simulink model "model"  (R2023a)
settings: Solver=VariableStepAuto  StartTime=0.0  StopTime=10.0  RelTol=1e-3
libraries: BatteryCurrentManagement x2
settings Model: Creator=Pedro  LastModifiedBy=Pedro

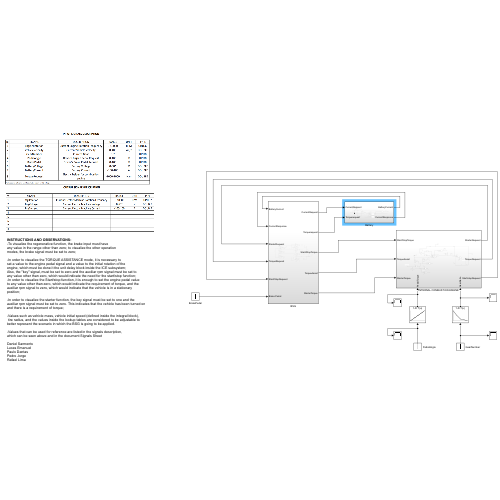
[thumbnail: Simulink's stored preview of the top-level diagram]
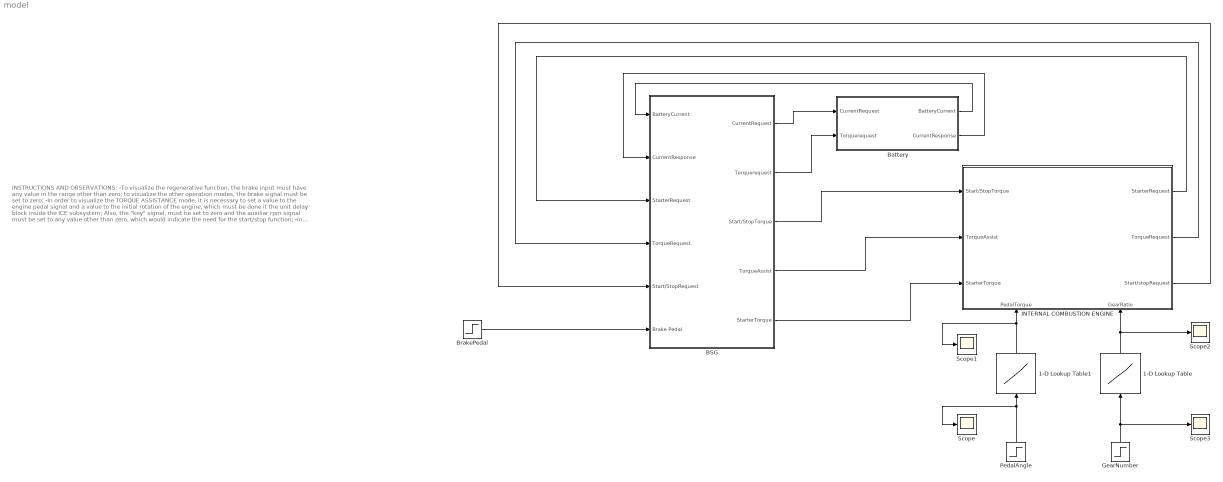
== system model ==
  note: INSTRUCTIONS AND OBSERVATIONS:
      | -To visualize the regenerative function, the brake input must have
      | any value in the range other than zero; to visualize the other operation
      | modes, the brake signal must be set to zero;
      |
      | -In order to visualize the TORQUE ASSISTANCE mode, it is necessary to
      | set a value to the engine pedal signal and a value to the initial rotation of the
      | engine, which must be done it the unit delay block inside the ICE subsystem;
      | Also, the "key" signal, must be set to zero and the auxiliar rpm signal must be set to
      | any value other than zero, which would indicate the need for the start/stop function;
      | -In order to visualize the Start/stop function, it is enough to set the engine pedal value
      | to any value other than zero, which would indicate the requirement of torque, and the
      | auxiliar rpm signal to zero, which would indicate that the vehicle is in a stationary
      | position;
      |
      | -In order to visualize the starter function, the key signal must be set to one and the
      | auxiliar rpm signal must be set to zero. This indicates that the vehicle has been turned on
      | and there is a requirement of torque;
      |
      | -Values such as vehicle mass, vehicle initial speed (defined inside the integral block),
      | tire radius, and the values inside the lookup tables are considered to be adjustable to
      | better represent the scenario in which the BSG is going to be applied.
      |
      | -Values that can be used for reference are listed in the signals description,
      | which can be seen above and in the document Signals Sheet
      |
      | Daniel Sarmento
      | Lucas Emanuel
      | Paulo Dantas
      | Pedro Jorge
      | Rafael Lima
  1-D Lookup Table : Lookup_n-D  NumberOfTableDimensions=1  BreakpointsForDimension1=[1 2 3 4 5]  Table=[3 2 1.2 1 0.8]  InternalRulePriority=Speed  RndMeth=Simplest
  1-D Lookup Table1 : Lookup_n-D  NumberOfTableDimensions=1  BreakpointsForDimension1=|  Table=|  InternalRulePriority=Speed  RndMeth=Simplest
      BreakpointsForDimension1=|
      | [0
      | 0.5
      | 1
      | 1.5
      | 2
      | 2.5
      | 3
      | 3.5
      | 4
      | 4.5
      | 5
      | 5.5
      | 6
      | 6.5
      | 7
      | 7.5
      | 8
      | 8.5
      | 9
      | 9.5
      | 10
      | 10.5
      | 11
      | 11.5
      | 12
      | 12.5
      | 13
      | 13.5
      | 14
      | 14.5
      | 15
      | 15.5
      | 16
      | 16.5
      | 17
      | 17.5
      | 18
      | 18.5
      | 19
      | 19.5
      | 20
      | 20.5
      | 21
      | 21.5
      | 22
      | 22.5
      | 23
      | 23.5
      | 24
      | 24.5
      | 25
      | 25.5
      | 26
      | 26.5
      | 27
      | 27.5
      | 28
      | 28.5
      | 29
      | 29.5
      | 30
      | 30.5
      | 31
      | 31.5
      | 32
      | 32.5
      | 33
      | 33.5
      | 34
      | 34.5
      | 35
      | 35.5
      | 36
      | 36.5
      | 37
      | 37.5
      | 38
      | 38.5
      | 39
      | 39.5
      | 40
      | 40.5
      | 41
      | 41.5
      | 42
      | 42.5
      | 43
      | 43.5
      | 44
      | 44.5
      | 45
      | 45.5
      | 46
      | 46.5
      | 47
      | 47.5
      | 48
      | 48.5
      | 49
      | 49.5
      | 50
      | 50.5
      | 51
      | 51.5
      | 52
      | 52.5
      | 53
      | 53.5
      | 54
      | 54.5
      | 55
      | 55.5
      | 56
      | 56.5
      | 57
      | 57.5
      | 58
      | 58.5
      | 59
      | 59.5
      | 60
      | 60.5
      | 61
      | 61.5
      | 62
      | 62.5
      | 63
      | 63.5
      | 64
      | 64.5
      | 65
      | 65.5
      | 66
      | 66.5
      | 67
      | 67.5
      | 68
      | 68.5
      | 69
      | 69.5
      | 70
      | 70.5
      | 71
      | 71.5
      | 72
      | 72.5
      | 73
      | 73.5
      | 74
      | 74.5
      | 75
      | 75.5
      | 76
      | 76.5
      | 77
      | 77.5
      | 78
      | 78.5
      | 79
      | 79.5
      | 80
      | 80.5
      | 81
      | 81.5
      | 82
      | 82.5
      | 83
      | 83.5
      | 84
      | 84.5
      | 85
      | 85.5
      | 86
      | 86.5
      | 87
      | 87.5
      | 88
      | 88.5
      | 89
      | 89.5
      | 90
      | 90.5
      | 91
      | 91.5
      | 92
      | 92.5
      | 93
      | 93.5
      | 94
      | 94.5
      | 95
      | 95.5
      | 96
      | 96.5
      | 97
      | 97.5
      | 98
      | 98.5
      | 99
      | 99.5
      | 100
      | ]
      Table=|
      | [0
      | 2
      | 4
      | 6
      | 8
      | 10
      | 12
      | 14
      | 16
      | 18
      | 20
      | 22
      | 24
      | 26
      | 28
      | 30
      | 32
      | 34
      | 36
      | 38
      | 40
      | 42
      | 44
      | 46
      | 48
      | 50
      | 52
      | 54
      | 56
      | 58
      | 60
      | 62
      | 64
      | 66
      | 68
      | 70
      | 72
      | 74
      | 76
      | 78
      | 80
      | 82
      | 84
      | 86
      | 88
      | 90
      | 92
      | 94
      | 96
      | 98
      | 100
      | 102
      | 104
      | 106
      | 108
      | 110
      | 112
      | 114
      | 116
      | 118
      | 120
      | 122
      | 124
      | 126
      | 128
      | 130
      | 132
      | 134
      | 136
      | 138
      | 140
      | 142
      | 144
      | 146
      | 148
      | 150
      | 152
      | 154
      | 156
      | 158
      | 160
      | 162
      | 164
      | 166
      | 168
      | 170
      | 172
      | 174
      | 176
      | 178
      | 180
      | 182
      | 184
      | 186
      | 188
      | 190
      | 192
      | 194
      | 196
      | 198
      | 200
      | 202
      | 204
      | 206
      | 208
      | 210
      | 212
      | 214
      | 216
      | 218
      | 220
      | 222
      | 224
      | 226
      | 228
      | 230
      | 232
      | 234
      | 236
      | 238
      | 240
      | 242
      | 244
      | 246
      | 248
      | 250
      | 252
      | 254
      | 256
      | 258
      | 260
      | 262
      | 264
      | 266
      | 268
      | 270
      | 272
      | 274
      | 276
      | 278
      | 280
      | 282
      | 284
      | 286
      | 288
      | 290
      | 292
      | 294
      | 296
      | 298
      | 300
      | 302
      | 304
      | 306
      | 308
      | 310
      | 312
      | 314
      | 316
      | 318
      | 320
      | 322
      | 324
      | 326
      | 328
      | 330
      | 332
      | 334
      | 336
      | 338
      | 340
      | 342
      | 344
      | 346
      | 348
      | 350
      | 352
      | 354
      | 356
      | 358
      | 360
      | 362
      | 364
      | 366
      | 368
      | 370
      | 372
      | 374
      | 376
      | 378
      | 380
      | 382
      | 384
      | 386
      | 388
      | 390
      | 392
      | 394
      | 396
      | 398
      | 400]
  BSG : Subsystem
  Battery : Subsystem
  BrakePedal : Step  Before=5  After=5  SampleTime=0
  GearNumber : Step  Before=3  After=3  SampleTime=0
  INTERNAL COMBUSTION ENGINE : Subsystem
      settings: PortSchema="{\"entries\":[{\"content\":{\"sides\":[{\"content\":{\"connectorIds\":[\"In1\",\"In2\",\"In3\"]},\"type\":\"ConnectorPlacement.EquallySpacedRectSide\",\"uuid\":\"ce092393-4b5e-4455-aba9-0cf9705a5882\"},{\"content\":{\"connectorIds\":[\"Out1\",\"Out2\",\"Out3\"],\"side\":\"RIGHT\"},\"type\":\"ConnectorPlacement.EquallySpacedRectSide\",\"uuid\":\"39f1620d-f19f-4d17-9a2c-1204b4040c22\"},{\"content\":{\"side\":\"TOP\"},\"type\":\"ConnectorPlacement.EquallySpacedRectSide\",\"uuid\":\"940edc2a-8e4d-4800-9ba5-7e24d0f8ee78\"},{\"content\":{\"connectorIds\":[\"In4\",\"In5\"],\"side\":\"BOTTOM\"},\"type\":\"ConnectorPlacement.EquallySpacedRectSide\",\"uuid\":\"a8c92029-a525-4a44-9138-e7028dc0182e\"}]},\"type\":\"ConnectorPlacement.EquallySpacedConnector\",\"uuid\":\"b09c41f2-a1e2-4cd1-915a-dc8e84f252cd\"}],\"packageUris\":[\"http://schema.mathworks.com/mf0/Connector/R2020b\"],\"version\":\"1.0\"}"
  PedalAngle : Step  Before=10  After=10  SampleTime=0
  Scope{,1..3} (4 alike) : Scope
  wires:
  Battery/2(CurrentResponse) -> BSG/2(CurrentResponse)
  PedalAngle/1 -> Scope/1, 1-D Lookup Table1/1
  BrakePedal/1 -> BSG/6(Brake Pedal)
  INTERNAL COMBUSTION ENGINE/2(TorqueRequest) -> BSG/4(TorqueRequest)
  INTERNAL COMBUSTION ENGINE/3(Start/stopRequest) -> BSG/5(Start/StopRequest)
  INTERNAL COMBUSTION ENGINE/1(StarterRequest) -> BSG/3(StarterRequest)
  GearNumber/1 -> 1-D Lookup Table/1, Scope3/1
  1-D Lookup Table/1 -> Scope2/1, INTERNAL COMBUSTION ENGINE/5(GearRatio)
  BSG/3(Start/StopTorque) -> INTERNAL COMBUSTION ENGINE/1(Start/StopTorque)
  BSG/4(TorqueAssist) -> INTERNAL COMBUSTION ENGINE/2(TorqueAssist)
  BSG/5(StarterTorque) -> INTERNAL COMBUSTION ENGINE/3(StarterTorque)
  Battery/1(BatteryCurrent) -> BSG/1(BatteryCurrent)
  BSG/1(CurrentRequest) -> Battery/1(CurrentRequest)
  1-D Lookup Table1/1 -> Scope1/1, INTERNAL COMBUSTION ENGINE/4(PedalTorque)
  BSG/2(Torquerequest) -> Battery/2(Torquerequest)

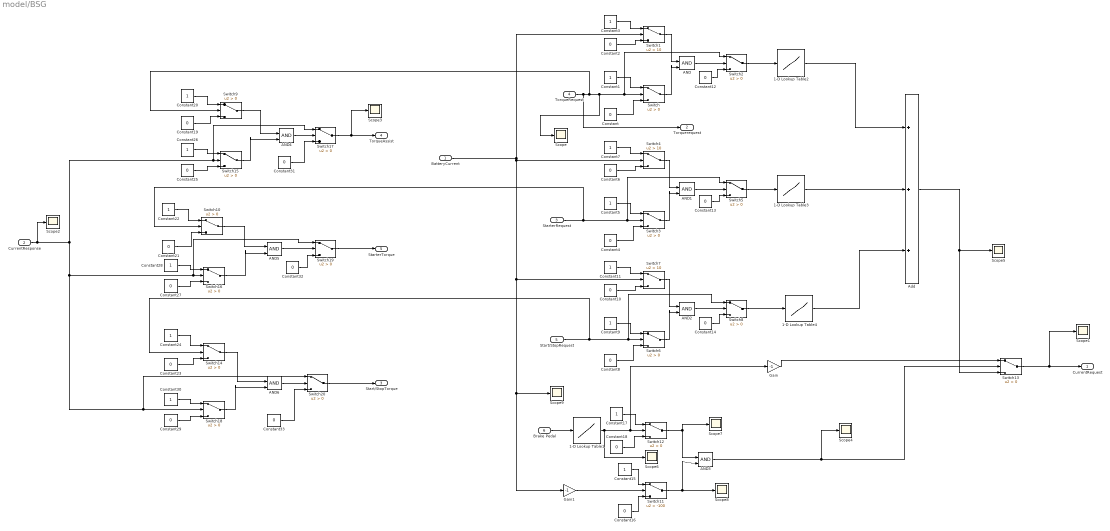
== system model/BSG ==
  BatteryCurrent : Inport
  CurrentResponse : Inport  Port=2
  StarterRequest : Inport  Port=3
  TorqueRequest : Inport  Port=4
  Start/StopRequest : Inport  Port=5
  Brake Pedal : Inport  Port=6
  1-D Lookup Table1 : Lookup_n-D  NumberOfTableDimensions=1  BreakpointsForDimension1=|  Table=|  InternalRulePriority=Speed  RndMeth=Simplest
      | [0
      | 5
      | 10
      | 15
      | 20
      | 25
      | 30
      | 35
      | 40
      | 45
      | 50
      | 55
      | 60
      | 65
      | 70
      | 75
      | 80
      | 85
      | 90
      | 95
      | 100
      | ]
      | [0
      | 5
      | 10
      | 15
      | 20
      | 25
      | 30
      | 35
      | 40
      | 45
      | 50
      | 55
      | 60
      | 65
      | 70
      | 75
      | 80
      | 85
      | 90
      | 95
      | 100
      | ]
  1-D Lookup Table2 : Lookup_n-D  NumberOfTableDimensions=1  BreakpointsForDimension1=|  Table=|  InternalRulePriority=Speed  RndMeth=Simplest
      | [0
      | 10
      | 20
      | 30
      | 40
      | 50
      | 60
      | 70
      | 80
      | 90
      | 100
      | 110
      | 120
      | 130
      | 140
      | 150
      | 160
      | 170
      | 180
      | 190
      | 200
      | 210
      | 220
      | 230
      | 240
      | 250
      | 260
      | 270
      | 280
      | 290
      | 300
      | ]
      | [0
      | 1.7
      | 4.4
      | 7.1
      | 9.8
      | 12.5
      | 15.2
      | 17.9
      | 20.6
      | 23.3
      | 26
      | 28.7
      | 31.4
      | 34.1
      | 36.8
      | 39.5
      | 42.2
      | 44.9
      | 47.6
      | 50.3
      | 53
      | 55.7
      | 58.4
      | 61.1
      | 63.8
      | 66.5
      | 69.2
      | 71.9
      | 74.6
      | 77.3
      | 80
      | ]
  1-D Lookup Table3 : Lookup_n-D  NumberOfTableDimensions=1  BreakpointsForDimension1=|  Table=|  InternalRulePriority=Speed  RndMeth=Simplest
      | [0
      | 10
      | 20
      | 30
      | 40
      | 50
      | 60
      | 70
      | 80
      | 90
      | 100
      | 110
      | 120
      | 130
      | 140
      | 150
      | 160
      | 170
      | 180
      | 190
      | 200
      | 210
      | 220
      | 230
      | 240
      | 250
      | 260
      | 270
      | 280
      | 290
      | 300
      | ]
      | [0
      | 1.7
      | 4.4
      | 7.1
      | 9.8
      | 12.5
      | 15.2
      | 17.9
      | 20.6
      | 23.3
      | 26
      | 28.7
      | 31.4
      | 34.1
      | 36.8
      | 39.5
      | 42.2
      | 44.9
      | 47.6
      | 50.3
      | 53
      | 55.7
      | 58.4
      | 61.1
      | 63.8
      | 66.5
      | 69.2
      | 71.9
      | 74.6
      | 77.3
      | 80
      | ]
  1-D Lookup Table4 : Lookup_n-D  NumberOfTableDimensions=1  BreakpointsForDimension1=|  Table=|  InternalRulePriority=Speed  RndMeth=Simplest
      | [0
      | 10
      | 20
      | 30
      | 40
      | 50
      | 60
      | 70
      | 80
      | 90
      | 100
      | 110
      | 120
      | 130
      | 140
      | 150
      | 160
      | 170
      | 180
      | 190
      | 200
      | 210
      | 220
      | 230
      | 240
      | 250
      | 260
      | 270
      | 280
      | 290
      | 300
      | ]
      | [0
      | 1.7
      | 4.4
      | 7.1
      | 9.8
      | 12.5
      | 15.2
      | 17.9
      | 20.6
      | 23.3
      | 26
      | 28.7
      | 31.4
      | 34.1
      | 36.8
      | 39.5
      | 42.2
      | 44.9
      | 47.6
      | 50.3
      | 53
      | 55.7
      | 58.4
      | 61.1
      | 63.8
      | 66.5
      | 69.2
      | 71.9
      | 74.6
      | 77.3
      | 80
      | ]
  AND{,1..6} (7 alike) : Logic  IconShape=distinctive  AllPortsSameDT=off  OutDataTypeStr=boolean
  Add : Sum  Inputs=+++
  Constant{,2,4,6,8,10,12..14,16,18..19,21,23,25,27,29,31..33} (20 alike) : Constant  Value=0
  Constant{1,3,5,7,9,11,15,17,20,22,24,26,28,30} (14 alike) : Constant
  Gain : Gain  Gain=-1
  Gain1 : Gain  Gain=-1
  Scope{,1..9} (10 alike) : Scope
  Switch{,2..3,5..6,8..10,12..20} (17 alike) : Switch  Criteria=u2 > Threshold  SaturateOnIntegerOverflow=off  InputSameDT=off
  Switch1 : Switch  Criteria=u2 > Threshold  Threshold=10  SaturateOnIntegerOverflow=off  InputSameDT=off
  Switch11 : Switch  Criteria=u2 > Threshold  Threshold=-100  SaturateOnIntegerOverflow=off  InputSameDT=off
  Switch4 : Switch  Criteria=u2 > Threshold  Threshold=10  SaturateOnIntegerOverflow=off  InputSameDT=off
  Switch7 : Switch  Criteria=u2 > Threshold  Threshold=10  SaturateOnIntegerOverflow=off  InputSameDT=off
  CurrentRequest : Outport
  Torquerequest : Outport  Port=2
  Start/StopTorque : Outport  Port=3
  TorqueAssist : Outport  Port=4
  StarterTorque : Outport  Port=5
  wires:
  Constant14/1 -> Switch8/3
  Constant11/1 -> Switch7/1
  Constant8/1 -> Switch6/3
  Constant6/1 -> Switch4/3
  Constant10/1 -> Switch7/3
  AND1/1 -> Switch5/2
  Constant12/1 -> Switch2/3
  Switch7/1 -> AND2/1
  StarterRequest/1 -> Switch10/2, Switch5/1, Switch3/2
  Constant13/1 -> Switch5/3
  AND2/1 -> Switch8/2
  AND/1 -> Switch2/2
  Constant4/1 -> Switch3/3
  Constant2/1 -> Switch1/3
  Constant5/1 -> Switch3/1
  Switch6/1 -> AND2/2
  Switch4/1 -> AND1/1
  Constant3/1 -> Switch1/1
  Constant/1 -> Switch/3
  Switch/1 -> AND/2
  1-D Lookup Table2/1 -> Add/1
  Constant1/1 -> Switch/1
  Switch3/1 -> AND1/2
  Switch5/1 -> 1-D Lookup Table3/1
  TorqueRequest/1 -> Torquerequest/1, Switch9/2, Scope/1, Switch2/1, Switch/2
  Start/StopRequest/1 -> Switch14/2, Switch8/1, Switch6/2
  Constant7/1 -> Switch4/1
  Constant9/1 -> Switch6/1
  BatteryCurrent/1 -> Gain1/1, Scope9/1, Switch7/2, Switch4/2, Switch1/2
  Switch2/1 -> 1-D Lookup Table2/1
  Switch1/1 -> AND/1
  Switch8/1 -> 1-D Lookup Table4/1
  Brake Pedal/1 -> 1-D Lookup Table1/1
  Constant15/1 -> Switch11/1
  Constant16/1 -> Switch11/3
  Gain1/1 -> Switch11/2
  1-D Lookup Table1/1 -> Scope6/1, Gain/1, Switch12/2
  Constant17/1 -> Switch12/1
  Constant18/1 -> Switch12/3
  Switch12/1 -> AND3/1, Scope7/1
  Switch11/1 -> AND3/2, Scope8/1
  Gain/1 -> Switch13/1
  1-D Lookup Table3/1 -> Add/2
  1-D Lookup Table4/1 -> Add/3
  Add/1 -> Switch13/3, Scope5/1
  Switch13/1 -> Scope1/1, CurrentRequest/1
  Constant19/1 -> Switch9/3
  Constant20/1 -> Switch9/1
  Constant22/1 -> Switch10/1
  Constant21/1 -> Switch10/3
  Constant23/1 -> Switch14/3
  Constant24/1 -> Switch14/1
  Constant25/1 -> Switch15/3
  CurrentResponse/1 -> Scope2/1, Switch20/1, Switch18/2, Switch19/1, Switch16/2, Switch17/1, Switch15/2
  Constant26/1 -> Switch15/1
  Constant27/1 -> Switch16/3
  Constant28/1 -> Switch16/1
  Constant29/1 -> Switch18/3
  Constant30/1 -> Switch18/1
  Switch9/1 -> AND4/1
  Switch15/1 -> AND4/2
  Switch10/1 -> AND5/1
  Switch16/1 -> AND5/2
  Switch14/1 -> AND6/1
  Switch18/1 -> AND6/2
  AND4/1 -> Switch17/2
  Constant31/1 -> Switch17/3
  AND5/1 -> Switch19/2
  Constant32/1 -> Switch19/3
  AND6/1 -> Switch20/2
  Constant33/1 -> Switch20/3
  Switch17/1 -> Scope3/1, TorqueAssist/1
  Switch19/1 -> StarterTorque/1
  Switch20/1 -> Start/StopTorque/1
  AND3/1 -> Scope4/1, Switch13/2

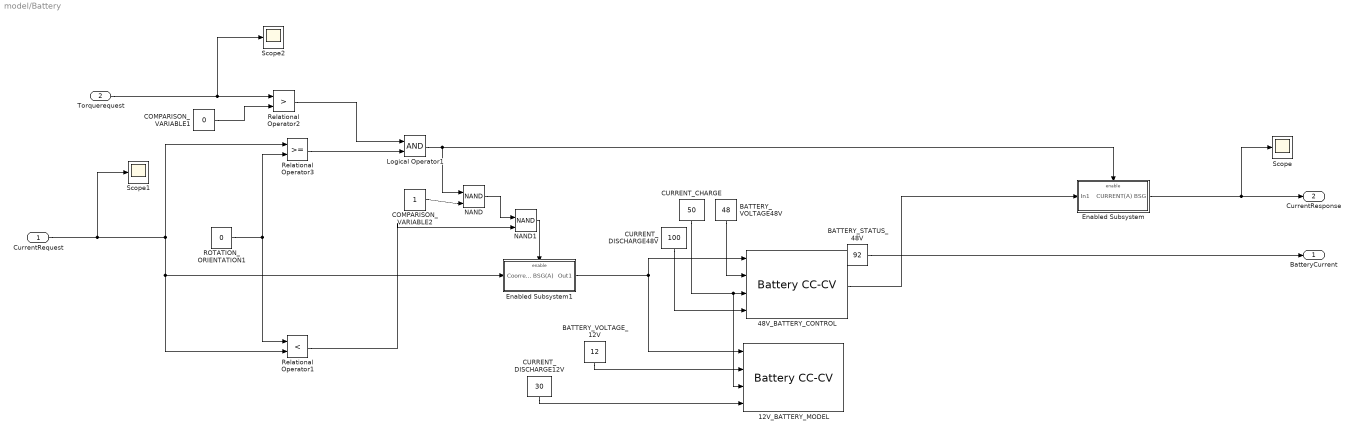
== system model/Battery ==
  CurrentRequest : Inport
  Torquerequest : Inport  Port=2
  12V_BATTERY_MODEL : BatteryCurrentManagement/Battery CC-CV  MaxCellVoltage=12  Kp=100  Ki=10  Kaw=1  Kt=1  Ts=1
      settings: LibrarySourceBlock=batt_sl_lib/Current Management/Battery CC-CV
  48V_BATTERY_CONTROL : BatteryCurrentManagement/Battery CC-CV  MaxCellVoltage=48  Kp=100  Ki=30  Kaw=1  Kt=1  Ts=1
      settings: LibrarySourceBlock=batt_sl_lib/Current Management/Battery CC-CV
  BATTERY_STATUS_48V : Constant  Value=92
  BATTERY_VOLTAGE48V : Constant  Value=48
  BATTERY_VOLTAGE_12V : Constant  Value=12
  COMPARISON_VARIABLE1 : Constant  Value=0
  COMPARISON_VARIABLE2 : Constant
  CURRENT_CHARGE : Constant  Value=50
  CURRENT_DISCHARGE12V : Constant  Value=30
  CURRENT_DISCHARGE48V : Constant  Value=100
  Enabled Subsystem : Subsystem  TreatAsAtomicUnit=on
  Enabled Subsystem1 : Subsystem  TreatAsAtomicUnit=on
  Logical Operator1 : Logic  AllPortsSameDT=off  OutDataTypeStr=boolean
  NAND : Logic  Operator=NAND  IconShape=distinctive  AllPortsSameDT=off  OutDataTypeStr=boolean
  NAND1 : Logic  Operator=NAND  IconShape=distinctive  AllPortsSameDT=off  OutDataTypeStr=boolean
  ROTATION_ORIENTATION1 : Constant  Value=0
  Relational Operator1 : RelationalOperator  Operator=<  OutDataTypeStr=boolean  RndMeth=Simplest  InputSameDT=off
  Relational Operator2 : RelationalOperator  Operator=>  OutDataTypeStr=boolean  RndMeth=Simplest  InputSameDT=off
  Relational Operator3 : RelationalOperator  OutDataTypeStr=boolean  RndMeth=Simplest  InputSameDT=off
  Scope : Scope
  Scope1 : Scope
  Scope2 : Scope
  BatteryCurrent : Outport
  CurrentResponse : Outport  Port=2
  wires:
  CURRENT_DISCHARGE48V/1 -> 48V_BATTERY_CONTROL/4
  Logical Operator1/1 -> NAND/1, Enabled Subsystem/Enable
  CURRENT_CHARGE/1 -> 12V_BATTERY_MODEL/3, 48V_BATTERY_CONTROL/3
  COMPARISON_VARIABLE1/1 -> Relational Operator2/2
  Enabled Subsystem1/1(Out1) -> 12V_BATTERY_MODEL/1, 48V_BATTERY_CONTROL/1
  Enabled Subsystem/1(CURRENT(A) BSG) -> Scope/1, CurrentResponse/1
  CurrentRequest/1 -> Enabled Subsystem1/1(Coorrente BSG(A)), Relational Operator1/2, Relational Operator3/1, Scope1/1
  Torquerequest/1 -> Scope2/1, Relational Operator2/1
  CURRENT_DISCHARGE12V/1 -> 12V_BATTERY_MODEL/4
  ROTATION_ORIENTATION1/1 -> Relational Operator3/2, Relational Operator1/1
  48V_BATTERY_CONTROL/1 -> Enabled Subsystem/1(In1)
  NAND/1 -> NAND1/1
  NAND1/1 -> Enabled Subsystem1/Enable
  Relational Operator1/1 -> NAND1/2
  COMPARISON_VARIABLE2/1 -> NAND/2
  BATTERY_VOLTAGE48V/1 -> 48V_BATTERY_CONTROL/2
  BATTERY_VOLTAGE_12V/1 -> 12V_BATTERY_MODEL/2
  Relational Operator3/1 -> Logical Operator1/2
  BATTERY_STATUS_48V/1 -> BatteryCurrent/1
  Relational Operator2/1 -> Logical Operator1/1

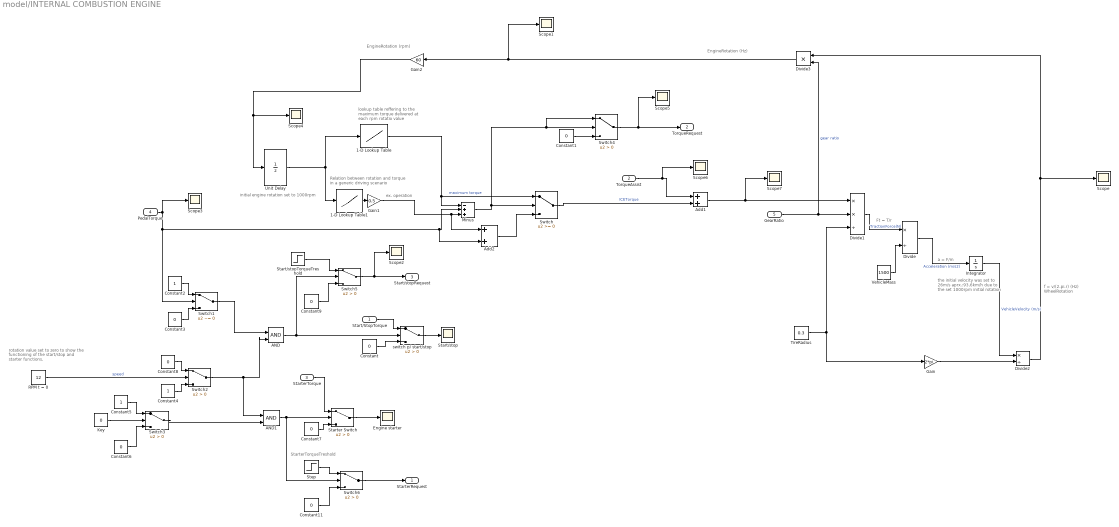
== system model/INTERNAL COMBUSTION ENGINE ==
  note: Relation between rotation and
      | torque in a generic driving scenario
  note: lookup table reffering to the
      | maximum torque delivered at
      | each rpm rotatio value
  note: rotation value set to zero to show
      | the functioning of the start/stop and
      | starter functions.
  note: StarterTorqueTreshold
  note: the initial velocity was set to
      | 26m/s aprx.:93,6km/h due to
      | the set 1000rpm initial rotation
  note: initial engine rotation set to 1000rpm
  note: EngineRotation (Hz)
  note: EngineRotation (rpm)
  note: ex. operation
  note: a = F/m
  note: f = v/(2.pi.r) (Hz)
      | WheelRotation
  note: Ft = T/r
  Start/StopTorque : Inport
  TorqueAssist : Inport  Port=2
  StarterTorque : Inport  Port=3
  PedalTorque : Inport  Port=4
  GearRatio : Inport  Port=5
  1-D Lookup Table : Lookup_n-D  NumberOfTableDimensions=1  BreakpointsForDimension1=[50;100;150;200;250;300;350;400;450;500;550;600;650;700;750;800;850;900;950;1000;1050;1100;1150;1200;1250;1300;1350;1400;1450;1500;1550;1600;1650;1700;1750;1800;1850;1900;1950;2000;2050;2100;2150;2200;2250;2300;2350;2400;2450;2500;2550;2600;2650;2700;2750;2800;2850;2900;2950;3000;3050;3100;3150;3200;3250;3300;3350;3400;3450;3500;3550;3600;3650;3700;3750;3800;3850;3900;3950;4000;4050;4100;4150;4200;4250;4300;4350;4400;4450;4500;4550;4600;4650;4700;4750;4800;4850;4900;4950;5000;5050;5100;5150;5200;5250;5300;5350;5400;5450;5500;5550;5600;5650;5700;5750;5800;5850;5900;5950;6000;6050;6100;6150;6200;6250;6300;6350;6400;6450;6500;6550;6600;6650;6700;6750;6800;6850;6900;6950;7000;7050;7100;7150;7200;7250;7300;7350;7400;7450;7500;7550;7600;7650;7700;7750;7800;7850;7900;7950;8000;8050;8100;8150;8200;8250;8300;8350;8400;8450;8500;8550;8600;8650;8700;8750;8800;8850;8900;8950;9000;9050;9100;9150;9200;9250;9300;9350;9400;9450;9500;9550;9600;9650;9700;9750;9800;9850;9900;9950;10000]  Table=[3;5;7;9;11;13;15;17;19;21;23;25;27;29;31;33;35;37;39;41;43;45;47;49;51;53;55;57;59;61;63;65;67;69;71;73;75;77;79;81;83;85;87;89;91;93;95;97;99;101;103;105;107;109;111;113;115;117;119;121;123;125;127;129;131;133;135;137;139;141;143;145;147;149;151;153;155;157;159;161;163;165;167;169;171;173;175;177;179;181;183;185;187;189;191;193;195;197;199;201;203;205;207;209;211;213;215;217;219;221;223;225;227;229;231;233;235;237;239;241;243;245;247;249;251;253;255;257;259;261;259;257;255;253;251;249;247;245;243;241;239;237;235;233;231;229;227;225;223;221;219;217;215;213;211;209;207;205;203;201;199;197;195;193;191;189;187;185;183;181;179;177;175;173;171;169;167;165;163;161;159;157;155;153;151;149;147;145;143;141;139;137;135;133;131;129;127;125;123;121]  InternalRulePriority=Speed  RndMeth=Simplest
  1-D Lookup Table1 : Lookup_n-D  NumberOfTableDimensions=1  BreakpointsForDimension1=[50;100;150;200;250;300;350;400;450;500;550;600;650;700;750;800;850;900;950;1000;1050;1100;1150;1200;1250;1300;1350;1400;1450;1500;1550;1600;1650;1700;1750;1800;1850;1900;1950;2000;2050;2100;2150;2200;2250;2300;2350;2400;2450;2500;2550;2600;2650;2700;2750;2800;2850;2900;2950;3000;3050;3100;3150;3200;3250;3300;3350;3400;3450;3500;3550;3600;3650;3700;3750;3800;3850;3900;3950;4000;4050;4100;4150;4200;4250;4300;4350;4400;4450;4500;4550;4600;4650;4700;4750;4800;4850;4900;4950;5000;5050;5100;5150;5200;5250;5300;5350;5400;5450;5500;5550;5600;5650;5700;5750;5800;5850;5900;5950;6000;6050;6100;6150;6200;6250;6300;6350;6400;6450;6500;6550;6600;6650;6700;6750;6800;6850;6900;6950;7000;7050;7100;7150;7200;7250;7300;7350;7400;7450;7500;7550;7600;7650;7700;7750;7800;7850;7900;7950;8000;8050;8100;8150;8200;8250;8300;8350;8400;8450;8500;8550;8600;8650;8700;8750;8800;8850;8900;8950;9000;9050;9100;9150;9200;9250;9300;9350;9400;9450;9500;9550;9600;9650;9700;9750;9800;9850;9900;9950;10000]  Table=[3;5;7;9;11;13;15;17;19;21;23;25;27;29;31;33;35;37;39;41;43;45;47;49;51;53;55;57;59;61;63;65;67;69;71;73;75;77;79;81;83;85;87;89;91;93;95;97;99;101;103;105;107;109;111;113;115;117;119;121;123;125;127;129;131;133;135;137;139;141;143;145;147;149;151;153;155;157;159;161;163;165;167;169;171;173;175;177;179;181;183;185;187;189;191;193;195;197;199;201;203;205;207;209;211;213;215;217;219;221;223;225;227;229;231;233;235;237;239;241;243;245;247;249;251;253;255;257;259;261;259;257;255;253;251;249;247;245;243;241;239;237;235;233;231;229;227;225;223;221;219;217;215;213;211;209;207;205;203;201;199;197;195;193;191;189;187;185;183;181;179;177;175;173;171;169;167;165;163;161;159;157;155;153;151;149;147;145;143;141;139;137;135;133;131;129;127;125;123;121]  InternalRulePriority=Speed  RndMeth=Simplest
  AND : Logic  IconShape=distinctive  AllPortsSameDT=off  OutDataTypeStr=boolean
  AND1 : Logic  IconShape=distinctive  AllPortsSameDT=off  OutDataTypeStr=boolean
  Add1 : Sum
  Add2 : Sum
  Constant{,1,3,6..9,11} (8 alike) : Constant  Value=0
  Constant2 : Constant
  Constant4 : Constant
  Constant5 : Constant
  Divide : Product  Inputs=*/
  Divide1 : Product  Inputs=**/
  Divide2 : Product  Inputs=*/
  Divide3 : Product  Inputs=**
  Engine starter : Scope
  Gain : Gain  Gain=2*pi
  Gain1 : Gain  Gain=0.5
  Gain2 : Gain  Gain=60
  Integrator : Integrator  InitialCondition=26
  Key : Constant  Value=0
  Minus : Sum  Inputs=-++
  RPM t = 0 : Constant  Value=12
  Scope{,1..7} (8 alike) : Scope
  Start/stop : Scope
  Start/stopTorqueTreshold : Step  SampleTime=0
  Starter Switch : Switch  Criteria=u2 > Threshold  SaturateOnIntegerOverflow=off  InputSameDT=off
  Step : Step  Before=70  After=70  SampleTime=0
  Switch : Switch  SaturateOnIntegerOverflow=off  InputSameDT=off
  Switch1 : Switch  Criteria=u2 ~= 0  SaturateOnIntegerOverflow=off  InputSameDT=off
  Switch{2..6} (5 alike) : Switch  Criteria=u2 > Threshold  SaturateOnIntegerOverflow=off  InputSameDT=off
  TireRadius : Constant  Value=0.3
  Unit Delay : UnitDelay  InitialCondition=1000  HasFrameUpgradeWarning=on
  VehicleMass : Constant  Value=1500
  switch p/ start/stop : Switch  Criteria=u2 > Threshold  SaturateOnIntegerOverflow=off  InputSameDT=off
  StarterRequest : Outport
  TorqueRequest : Outport  Port=2
  Start/stopRequest : Outport  Port=3
  wires:
  AND/1 -> Switch5/2, switch p/ start/stop/2
  RPM t = 0/1 -> Switch2/2  "speed"
  1-D Lookup Table/1 -> Switch/1, Minus/1  "maximum torque"
  PedalTorque/1 -> Scope3/1, Switch1/2, Add2/2, Minus/2
  Constant5/1 -> Switch3/1
  Constant2/1 -> Switch1/1
  Switch2/1 -> AND1/1, AND/2
  Constant3/1 -> Switch1/3
  Switch/1 -> Add1/2  "ICETorque"
  VehicleMass/1 -> Divide/2
  Minus/1 -> Switch4/1, Switch4/2, Switch/2
  Unit Delay/1 -> 1-D Lookup Table/1, 1-D Lookup Table1/1
  Start/StopTorque/1 -> switch p/ start/stop/1
  Constant/1 -> switch p/ start/stop/3
  Switch3/1 -> AND1/2
  Gain/1 -> Divide2/2
  Divide/1 -> Integrator/1  "Acceleration (m/s2)"
  TireRadius/1 -> Divide1/3, Gain/1
  Divide1/1 -> Divide/1  "TractionForce(N)"
  switch p/ start/stop/1 -> Start/stop/1
  Key/1 -> Switch3/2
  Integrator/1 -> Divide2/1  "VehicleVelocity (m/s)"
  AND1/1 -> Switch6/2, Starter Switch/2
  Constant6/1 -> Switch3/3
  Switch1/1 -> AND/1
  Constant4/1 -> Switch2/3
  Constant1/1 -> Switch4/3
  Switch4/1 -> Scope5/1, TorqueRequest/1
  TorqueAssist/1 -> Scope6/1, Add1/1
  Add1/1 -> Scope7/1, Divide1/1
  GearRatio/1 -> Divide3/2, Divide1/2  "gear ratio"
  StarterTorque/1 -> Starter Switch/1
  Constant7/1 -> Starter Switch/3
  Constant8/1 -> Switch2/1
  Starter Switch/1 -> Engine starter/1
  Start/stopTorqueTreshold/1 -> Switch5/1
  Constant9/1 -> Switch5/3
  Switch5/1 -> Scope2/1, Start/stopRequest/1
  Constant11/1 -> Switch6/3
  Switch6/1 -> StarterRequest/1
  Divide2/1 -> Divide3/1, Scope/1
  1-D Lookup Table1/1 -> Gain1/1
  Gain1/1 -> Add2/1, Minus/3
  Add2/1 -> Switch/3
  Divide3/1 -> Scope1/1, Gain2/1
  Gain2/1 -> Unit Delay/1, Scope4/1
  Step/1 -> Switch6/1

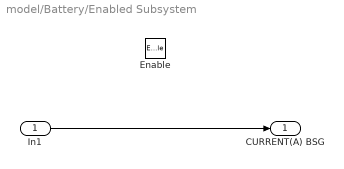
== system model/Battery/Enabled Subsystem ==
  In1 : Inport
  Enable : EnablePort
  CURRENT(A) BSG : Outport
  wires:
  In1/1 -> CURRENT(A) BSG/1

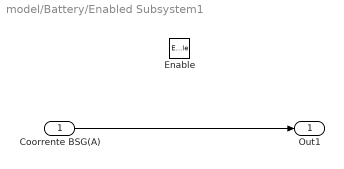
== system model/Battery/Enabled Subsystem1 ==
  Coorrente BSG(A) : Inport
  Enable : EnablePort
  Out1 : Outport
  wires:
  Coorrente BSG(A)/1 -> Out1/1
